simulink model "observer"  (R2017a)
settings: Solver=VariableStepAuto  StartTime=0.0  StopTime=30  RelTol=1e-3
values from neighbouring files (symbols this model uses):
  A = [-8.8487+(a-b)/5 -0.0399 -5.55+(c+d)/10 3.5846 ... (first row only)    [initialize.m]
  B = [0.0564+b/(10+c) 0.0319 ... (first row only)    [initialize.m]
  C = [-3.2988 -2.1932+(10*c+d)/(100+5*a) 0.037 -0.0109 ... (first row only)    [initialize.m]
  K_LQR = real(K_LQR)    [LQR.m]    (also in MIMO_servo_control_with_observer.m; MIMO_servo_control_without_observer.m; full_order_observer.m; last_task.m)
  L = transpose(K)    [MIMO_servo_control_with_observer.m]    (also in full_order_observer.m)
settings Model: Creator=lenovo  LastModifiedBy=lenovo

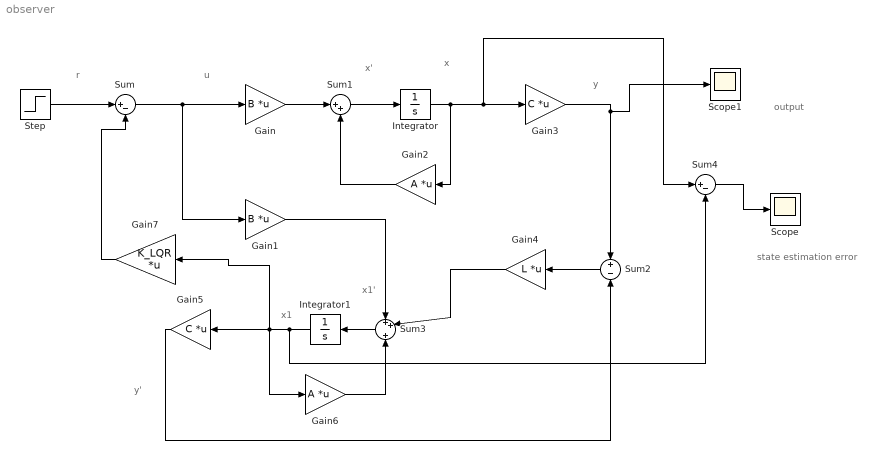
== system observer ==
  note: output
  note: state estimation error
  note: y'
  note: y
  note: x1'
  note: x1
  note: x
  note: x'
  note: u
  note: r
  Gain : Gain  Gain=B  Multiplication=Matrix(K*u)
  Gain1 : Gain  Gain=B  Multiplication=Matrix(K*u)
  Gain2 : Gain  Gain=A  Multiplication=Matrix(K*u)
  Gain3 : Gain  Gain=C  Multiplication=Matrix(K*u)
  Gain4 : Gain  Gain=L  Multiplication=Matrix(K*u)
  Gain5 : Gain  Gain=C  Multiplication=Matrix(K*u)
  Gain6 : Gain  Gain=A  Multiplication=Matrix(K*u)
  Gain7 : Gain  Gain=K_LQR  Multiplication=Matrix(K*u)
  Integrator : Integrator  InitialCondition=[0.5;-0.1;0.3;-0.8]
  Integrator1 : Integrator
  Scope : Scope
  Scope1 : Scope
  Step : Step  Before=[0;1]  After=[0;0]  SampleTime=0  VectorParams1D=off
  Sum : Sum  Inputs=|+-
  Sum1 : Sum  Inputs=|++
  Sum2 : Sum  Inputs=+|-
  Sum3 : Sum  Inputs=++|+
  Sum4 : Sum  Inputs=|+-
  wires:
  Gain/1 -> Sum1/1
  Gain2/1 -> Sum1/2
  Sum1/1 -> Integrator/1
  Gain3/1 -> Scope1/1, Sum2/1
  Sum2/1 -> Gain4/1
  Step/1 -> Sum/1
  Sum/1 -> Gain1/1, Gain/1
  Gain4/1 -> Sum3/2
  Gain1/1 -> Sum3/1
  Gain5/1 -> Sum2/2
  Sum3/1 -> Integrator1/1
  Gain6/1 -> Sum3/3
  Gain7/1 -> Sum/2
  Integrator/1 -> Sum4/1, Gain3/1, Gain2/1
  Integrator1/1 -> Sum4/2, Gain7/1, Gain6/1, Gain5/1
  Sum4/1 -> Scope/1
